simulink model "test_mdl_NI"  (R2018a)
settings: Solver=VariableStepAuto  StartTime=0.0  StopTime=10.0  RelTol=1e-3
(part 9 of 24)

== system test_mdl_NI/Subsystem/GWM/Body_Info_4_FD1_Ox242 ==
  in_port : Inport
  BattULo_I_Actl : Terminator
  BattULo_U_Actl : Terminator
  BrkTrnShifLck_B_Stat : Terminator
  DcacElPw_D_Rq : Terminator
  DriverCrankingReq : Terminator
  EngOff_T_Actl : Terminator
  FuelPumpPwr_D_Stat : Terminator
  PrkLckCtlAvail_T_Stat : Terminator
  PrkLckCtlMsgTxt_D_Rq : Terminator
  PrkLckCtlTow_B_Enbl : Terminator
  PrkLckCtlUnlck_D_Stat : Terminator
  PrkLckCtl_B_Enbl : Terminator
  PtLatchActv_B_RqBcm : Terminator
  ReFuelSwtchStat_D_Actl : Terminator
  bus_selector : BusSelector  OutputSignals=BattULo_I_Actl,BattULo_U_Actl,BrkTrnShifLck_B_Stat,DcacElPw_D_Rq,DriverCrankingReq,EngOff_T_Actl,FuelPumpPwr_D_Stat,PrkLckCtlAvail_T_Stat,PrkLckCtlMsgTxt_D_Rq,PrkLckCtlTow_B_Enbl,PrkLckCtlUnlck_D_Stat,PrkLckCtl_B_Enbl,PtLatchActv_B_RqBcm,ReFuelSwtchStat_D_Actl,immoSecureIdleMode
  immoSecureIdleMode : Terminator
  wires:
  in_port/1 -> bus_selector/1  "Body_Info_4_FD1_Ox242"
  bus_selector/1 -> BattULo_I_Actl/1  "<BattULo_I_Actl>"
  bus_selector/2 -> BattULo_U_Actl/1  "<BattULo_U_Actl>"
  bus_selector/3 -> BrkTrnShifLck_B_Stat/1  "<BrkTrnShifLck_B_Stat>"
  bus_selector/4 -> DcacElPw_D_Rq/1  "<DcacElPw_D_Rq>"
  bus_selector/5 -> DriverCrankingReq/1  "<DriverCrankingReq>"
  bus_selector/6 -> EngOff_T_Actl/1  "<EngOff_T_Actl>"
  bus_selector/7 -> FuelPumpPwr_D_Stat/1  "<FuelPumpPwr_D_Stat>"
  bus_selector/8 -> PrkLckCtlAvail_T_Stat/1  "<PrkLckCtlAvail_T_Stat>"
  bus_selector/9 -> PrkLckCtlMsgTxt_D_Rq/1  "<PrkLckCtlMsgTxt_D_Rq>"
  bus_selector/10 -> PrkLckCtlTow_B_Enbl/1  "<PrkLckCtlTow_B_Enbl>"
  bus_selector/11 -> PrkLckCtlUnlck_D_Stat/1  "<PrkLckCtlUnlck_D_Stat>"
  bus_selector/12 -> PrkLckCtl_B_Enbl/1  "<PrkLckCtl_B_Enbl>"
  bus_selector/13 -> PtLatchActv_B_RqBcm/1  "<PtLatchActv_B_RqBcm>"
  bus_selector/14 -> ReFuelSwtchStat_D_Actl/1  "<ReFuelSwtchStat_D_Actl>"
  bus_selector/15 -> immoSecureIdleMode/1  "<immoSecureIdleMode>"

== system test_mdl_NI/Subsystem/GWM/Body_Info_6_FD1_Ox38D ==
  in_port : Inport
  DrLatchMsgTxt_D_Rq : Terminator
  ElPwPoint_D_Rq : Terminator
  HeadLghtHiPrmsn_D_Stat : Terminator
  IgnPsswrdDsply_B_Rq : Terminator
  KeyAdmnTot_No_Cnt : Terminator
  KeyMykeyTot_No_Cnt : Terminator
  Keycode_Status : Terminator
  PEBackupSlot_Stats : Terminator
  PoliceIdlMde_D_Stat : Terminator
  PrmtrAlrmEvnt_D_Stat : Terminator
  PrsnlDevcChrgEnbl_B_Rq : Terminator
  SecurityMsgTxt_D_Rq : Terminator
  SteWhlLckMsgTxt_D_Rq : Terminator
  TracKeyMde_D_Stat : Terminator
  bus_selector : BusSelector  OutputSignals=DrLatchMsgTxt_D_Rq,ElPwPoint_D_Rq,HeadLghtHiPrmsn_D_Stat,IgnPsswrdDsply_B_Rq,KeyAdmnTot_No_Cnt,KeyMykeyTot_No_Cnt,Keycode_Status,PEBackupSlot_Stats,PoliceIdlMde_D_Stat,PrmtrAlrmEvnt_D_Stat,PrsnlDevcChrgEnbl_B_Rq,SecurityMsgTxt_D_Rq,SteWhlLckMsgTxt_D_Rq,TracKeyMde_D_Stat,immoMsgTxt_D_Rq
  immoMsgTxt_D_Rq : Terminator
  wires:
  in_port/1 -> bus_selector/1  "Body_Info_6_FD1_Ox38D"
  bus_selector/1 -> DrLatchMsgTxt_D_Rq/1  "<DrLatchMsgTxt_D_Rq>"
  bus_selector/2 -> ElPwPoint_D_Rq/1  "<ElPwPoint_D_Rq>"
  bus_selector/3 -> HeadLghtHiPrmsn_D_Stat/1  "<HeadLghtHiPrmsn_D_Stat>"
  bus_selector/4 -> IgnPsswrdDsply_B_Rq/1  "<IgnPsswrdDsply_B_Rq>"
  bus_selector/5 -> KeyAdmnTot_No_Cnt/1  "<KeyAdmnTot_No_Cnt>"
  bus_selector/6 -> KeyMykeyTot_No_Cnt/1  "<KeyMykeyTot_No_Cnt>"
  bus_selector/7 -> Keycode_Status/1  "<Keycode_Status>"
  bus_selector/8 -> PEBackupSlot_Stats/1  "<PEBackupSlot_Stats>"
  bus_selector/9 -> PoliceIdlMde_D_Stat/1  "<PoliceIdlMde_D_Stat>"
  bus_selector/10 -> PrmtrAlrmEvnt_D_Stat/1  "<PrmtrAlrmEvnt_D_Stat>"
  bus_selector/11 -> PrsnlDevcChrgEnbl_B_Rq/1  "<PrsnlDevcChrgEnbl_B_Rq>"
  bus_selector/12 -> SecurityMsgTxt_D_Rq/1  "<SecurityMsgTxt_D_Rq>"
  bus_selector/13 -> SteWhlLckMsgTxt_D_Rq/1  "<SteWhlLckMsgTxt_D_Rq>"
  bus_selector/14 -> TracKeyMde_D_Stat/1  "<TracKeyMde_D_Stat>"
  bus_selector/15 -> immoMsgTxt_D_Rq/1  "<immoMsgTxt_D_Rq>"

== system test_mdl_NI/Subsystem/GWM/Body_Info_8_FD1_Ox3B9 ==
  in_port : Inport
  BattRgenLoChrg_D_Rq : Terminator
  BattRgenLoDChrg_D_Rq : Terminator
  ChrgCordLck_B_Stat : Terminator
  ChrgCordResp1_No_Actl : Terminator
  ChrgCordResp2_No_Actl : Terminator
  WakeAlarm0_D_Stat : Terminator
  WakeAlarm1_D_Stat : Terminator
  WakeAlarm2_D_Stat : Terminator
  WakeAlarm3_D_Stat : Terminator
  bus_selector : BusSelector  OutputSignals=BattRgenLoChrg_D_Rq,BattRgenLoDChrg_D_Rq,ChrgCordLck_B_Stat,ChrgCordResp1_No_Actl,ChrgCordResp2_No_Actl,WakeAlarm0_D_Stat,WakeAlarm1_D_Stat,WakeAlarm2_D_Stat,WakeAlarm3_D_Stat
  wires:
  in_port/1 -> bus_selector/1  "Body_Info_8_FD1_Ox3B9"
  bus_selector/1 -> BattRgenLoChrg_D_Rq/1  "<BattRgenLoChrg_D_Rq>"
  bus_selector/2 -> BattRgenLoDChrg_D_Rq/1  "<BattRgenLoDChrg_D_Rq>"
  bus_selector/3 -> ChrgCordLck_B_Stat/1  "<ChrgCordLck_B_Stat>"
  bus_selector/4 -> ChrgCordResp1_No_Actl/1  "<ChrgCordResp1_No_Actl>"
  bus_selector/5 -> ChrgCordResp2_No_Actl/1  "<ChrgCordResp2_No_Actl>"
  bus_selector/6 -> WakeAlarm0_D_Stat/1  "<WakeAlarm0_D_Stat>"
  bus_selector/7 -> WakeAlarm1_D_Stat/1  "<WakeAlarm1_D_Stat>"
  bus_selector/8 -> WakeAlarm2_D_Stat/1  "<WakeAlarm2_D_Stat>"
  bus_selector/9 -> WakeAlarm3_D_Stat/1  "<WakeAlarm3_D_Stat>"

== system test_mdl_NI/Subsystem/GWM/Body_Info_9_FD1_Ox3A3 ==
  in_port : Inport
  AdvStrt_D_Stat : Terminator
  CrnkInhbt_B_Stat : Terminator
  CrnkInhbt_No_Cnt : Terminator
  CrnkInhbt_No_Cs : Terminator
  DrvInCtl_B_Stat : Terminator
  EngStrtActv_B_Stat : Terminator
  EngStrt_B_Rq : Terminator
  IgnPreOffActv_B_Stat : Terminator
  PtWakeReas_D_Stat : Terminator
  StrtrMtrCtlDStat_No_Cs : Terminator
  VehOnSrc_D_Stat : Terminator
  bus_selector : BusSelector  OutputSignals=AdvStrt_D_Stat,CrnkInhbt_B_Stat,CrnkInhbt_No_Cnt,CrnkInhbt_No_Cs,DrvInCtl_B_Stat,EngStrtActv_B_Stat,EngStrt_B_Rq,IgnPreOffActv_B_Stat,PtWakeReas_D_Stat,StrtrMtrCtlDStat_No_Cs,VehOnSrc_D_Stat
  wires:
  in_port/1 -> bus_selector/1  "Body_Info_9_FD1_Ox3A3"
  bus_selector/1 -> AdvStrt_D_Stat/1  "<AdvStrt_D_Stat>"
  bus_selector/2 -> CrnkInhbt_B_Stat/1  "<CrnkInhbt_B_Stat>"
  bus_selector/3 -> CrnkInhbt_No_Cnt/1  "<CrnkInhbt_No_Cnt>"
  bus_selector/4 -> CrnkInhbt_No_Cs/1  "<CrnkInhbt_No_Cs>"
  bus_selector/5 -> DrvInCtl_B_Stat/1  "<DrvInCtl_B_Stat>"
  bus_selector/6 -> EngStrtActv_B_Stat/1  "<EngStrtActv_B_Stat>"
  bus_selector/7 -> EngStrt_B_Rq/1  "<EngStrt_B_Rq>"
  bus_selector/8 -> IgnPreOffActv_B_Stat/1  "<IgnPreOffActv_B_Stat>"
  bus_selector/9 -> PtWakeReas_D_Stat/1  "<PtWakeReas_D_Stat>"
  bus_selector/10 -> StrtrMtrCtlDStat_No_Cs/1  "<StrtrMtrCtlDStat_No_Cs>"
  bus_selector/11 -> VehOnSrc_D_Stat/1  "<VehOnSrc_D_Stat>"

== system test_mdl_NI/Subsystem/GWM/Climate_Cntrl_Data_2_FD1_Ox35E ==
  in_port : Inport
  AutoStpHvacDelta_I_Est : Terminator
  CabnAmb_Te_Actl : Terminator
  ClimtThrmlLoad_No_Actl : Terminator
  HvacAir_Flw_Est : Terminator
  HvacBlwrFront_D_Stat : Terminator
  HvacRec_Pc_Est : Terminator
  HvacRemoteStrt_N_Rq : Terminator
  bus_selector : BusSelector  OutputSignals=AutoStpHvacDelta_I_Est,CabnAmb_Te_Actl,ClimtThrmlLoad_No_Actl,HvacAir_Flw_Est,HvacBlwrFront_D_Stat,HvacRec_Pc_Est,HvacRemoteStrt_N_Rq
  wires:
  in_port/1 -> bus_selector/1  "Climate_Cntrl_Data_2_FD1_Ox35E"
  bus_selector/1 -> AutoStpHvacDelta_I_Est/1  "<AutoStpHvacDelta_I_Est>"
  bus_selector/2 -> CabnAmb_Te_Actl/1  "<CabnAmb_Te_Actl>"
  bus_selector/3 -> ClimtThrmlLoad_No_Actl/1  "<ClimtThrmlLoad_No_Actl>"
  bus_selector/4 -> HvacAir_Flw_Est/1  "<HvacAir_Flw_Est>"
  bus_selector/5 -> HvacBlwrFront_D_Stat/1  "<HvacBlwrFront_D_Stat>"
  bus_selector/6 -> HvacRec_Pc_Est/1  "<HvacRec_Pc_Est>"
  bus_selector/7 -> HvacRemoteStrt_N_Rq/1  "<HvacRemoteStrt_N_Rq>"

== system test_mdl_NI/Subsystem/GWM/Climate_Control_Data_FD1_Ox41A ==
  in_port : Inport
  AutoHoldSwtch_D_Stat : Terminator
  LpdbDfrstRearOn_B_Rq : Terminator
  LpdbHeatWiprPrk_B_Rq : Terminator
  LpdbPtc1_B_Rq : Terminator
  LpdbPtc2_B_Rq : Terminator
  LpdbPtc3_B_Rq : Terminator
  MirrorHeatOn_B_Rq : Terminator
  Outside_Air_Temp_Stat : Terminator
  Remote_Start_QuietMode : Terminator
  SteWhlHeat_D_Rq : Terminator
  bus_selector : BusSelector  OutputSignals=AutoHoldSwtch_D_Stat,LpdbDfrstRearOn_B_Rq,LpdbHeatWiprPrk_B_Rq,LpdbPtc1_B_Rq,LpdbPtc2_B_Rq,LpdbPtc3_B_Rq,MirrorHeatOn_B_Rq,Outside_Air_Temp_Stat,Remote_Start_QuietMode,SteWhlHeat_D_Rq
  wires:
  in_port/1 -> bus_selector/1  "Climate_Control_Data_FD1_Ox41A"
  bus_selector/1 -> AutoHoldSwtch_D_Stat/1  "<AutoHoldSwtch_D_Stat>"
  bus_selector/2 -> LpdbDfrstRearOn_B_Rq/1  "<LpdbDfrstRearOn_B_Rq>"
  bus_selector/3 -> LpdbHeatWiprPrk_B_Rq/1  "<LpdbHeatWiprPrk_B_Rq>"
  bus_selector/4 -> LpdbPtc1_B_Rq/1  "<LpdbPtc1_B_Rq>"
  bus_selector/5 -> LpdbPtc2_B_Rq/1  "<LpdbPtc2_B_Rq>"
  bus_selector/6 -> LpdbPtc3_B_Rq/1  "<LpdbPtc3_B_Rq>"
  bus_selector/7 -> MirrorHeatOn_B_Rq/1  "<MirrorHeatOn_B_Rq>"
  bus_selector/8 -> Outside_Air_Temp_Stat/1  "<Outside_Air_Temp_Stat>"
  bus_selector/9 -> Remote_Start_QuietMode/1  "<Remote_Start_QuietMode>"
  bus_selector/10 -> SteWhlHeat_D_Rq/1  "<SteWhlHeat_D_Rq>"

== system test_mdl_NI/Subsystem/GWM/Cluster_HEV_Data8_FD1_Ox317 ==
  in_port : Inport
  ConsAvgTrip_Fe_Dsply : Terminator
  DrvEffLvl_No_Stat : Terminator
  EngAirFilt_B_RqReset : Terminator
  GpsElMdeSel_B_Rq : Terminator
  LongTermReset_B_Rq : Terminator
  bus_selector : BusSelector  OutputSignals=ConsAvgTrip_Fe_Dsply,DrvEffLvl_No_Stat,EngAirFilt_B_RqReset,GpsElMdeSel_B_Rq,LongTermReset_B_Rq
  wires:
  in_port/1 -> bus_selector/1  "Cluster_HEV_Data8_FD1_Ox317"
  bus_selector/1 -> ConsAvgTrip_Fe_Dsply/1  "<ConsAvgTrip_Fe_Dsply>"
  bus_selector/2 -> DrvEffLvl_No_Stat/1  "<DrvEffLvl_No_Stat>"
  bus_selector/3 -> EngAirFilt_B_RqReset/1  "<EngAirFilt_B_RqReset>"
  bus_selector/4 -> GpsElMdeSel_B_Rq/1  "<GpsElMdeSel_B_Rq>"
  bus_selector/5 -> LongTermReset_B_Rq/1  "<LongTermReset_B_Rq>"

== system test_mdl_NI/Subsystem/GWM/Cluster_Info1_FD1_Ox430 ==
  in_port : Inport
  AccDeny_B_RqIpc : Terminator
  AccEnbl_B_RqDrv : Terminator
  BulbChkActv_B_Stat : Terminator
  DrvSlipCtlMde_B_Rq2 : Terminator
  DrvSlipCtlMde_D_Rq : Terminator
  EngIdlShutDown_B_RqDrv : Terminator
  EngOilLife_B_RqReset : Terminator
  HaDsplyCpblty_B_Stat : Terminator
  HsaMde_D_Rq : Terminator
  KeyTypeChngMykey_D_Rq : Terminator
  LscmbbStat_B_Actl : Terminator
  ManRgen_D_Rq : Terminator
  MetricActv_B_Actl : Terminator
  NtrlTowMdeEnbl_B_RqDrv : Terminator
  OdometerMasterValue : Terminator
  ParkDetect_Stat : Terminator
  Power_Liftgate_Mode_Cmd : Terminator
  ReducedGuard_D_Rq : Terminator
  TRAILER_BRAKE_CONFIG : Terminator
  TRLR_SWAY_CONFIG_CMD : Terminator
  TrlrBrkMde_D_Rq : Terminator
  bus_selector : BusSelector  OutputSignals=AccDeny_B_RqIpc,AccEnbl_B_RqDrv,BulbChkActv_B_Stat,DrvSlipCtlMde_B_Rq2,DrvSlipCtlMde_D_Rq,EngIdlShutDown_B_RqDrv,EngOilLife_B_RqReset,HaDsplyCpblty_B_Stat,HsaMde_D_Rq,KeyTypeChngMykey_D_Rq,LscmbbStat_B_Actl,ManRgen_D_Rq,MetricActv_B_Actl,NtrlTowMdeEnbl_B_RqDrv,OdometerMasterValue,ParkDetect_Stat,Power_Liftgate_Mode_Cmd,ReducedGuard_D_Rq,TRAILER_BRAKE_CONFIG,TRLR_SWAY_CONFIG_CMD,TrlrBrkMde_D_Rq,ePRNDL_MODE
  ePRNDL_MODE : Terminator
  wires:
  in_port/1 -> bus_selector/1  "Cluster_Info1_FD1_Ox430"
  bus_selector/1 -> AccDeny_B_RqIpc/1  "<AccDeny_B_RqIpc>"
  bus_selector/2 -> AccEnbl_B_RqDrv/1  "<AccEnbl_B_RqDrv>"
  bus_selector/3 -> BulbChkActv_B_Stat/1  "<BulbChkActv_B_Stat>"
  bus_selector/4 -> DrvSlipCtlMde_B_Rq2/1  "<DrvSlipCtlMde_B_Rq2>"
  bus_selector/5 -> DrvSlipCtlMde_D_Rq/1  "<DrvSlipCtlMde_D_Rq>"
  bus_selector/6 -> EngIdlShutDown_B_RqDrv/1  "<EngIdlShutDown_B_RqDrv>"
  bus_selector/7 -> EngOilLife_B_RqReset/1  "<EngOilLife_B_RqReset>"
  bus_selector/8 -> HaDsplyCpblty_B_Stat/1  "<HaDsplyCpblty_B_Stat>"
  bus_selector/9 -> HsaMde_D_Rq/1  "<HsaMde_D_Rq>"
  bus_selector/10 -> KeyTypeChngMykey_D_Rq/1  "<KeyTypeChngMykey_D_Rq>"
  bus_selector/11 -> LscmbbStat_B_Actl/1  "<LscmbbStat_B_Actl>"
  bus_selector/12 -> ManRgen_D_Rq/1  "<ManRgen_D_Rq>"
  bus_selector/13 -> MetricActv_B_Actl/1  "<MetricActv_B_Actl>"
  bus_selector/14 -> NtrlTowMdeEnbl_B_RqDrv/1  "<NtrlTowMdeEnbl_B_RqDrv>"
  bus_selector/15 -> OdometerMasterValue/1  "<OdometerMasterValue>"
  bus_selector/16 -> ParkDetect_Stat/1  "<ParkDetect_Stat>"
  bus_selector/17 -> Power_Liftgate_Mode_Cmd/1  "<Power_Liftgate_Mode_Cmd>"
  bus_selector/18 -> ReducedGuard_D_Rq/1  "<ReducedGuard_D_Rq>"
  bus_selector/19 -> TRAILER_BRAKE_CONFIG/1  "<TRAILER_BRAKE_CONFIG>"
  bus_selector/20 -> TRLR_SWAY_CONFIG_CMD/1  "<TRLR_SWAY_CONFIG_CMD>"
  bus_selector/21 -> TrlrBrkMde_D_Rq/1  "<TrlrBrkMde_D_Rq>"
  bus_selector/22 -> ePRNDL_MODE/1  "<ePRNDL_MODE>"

== system test_mdl_NI/Subsystem/GWM/Cluster_Info_3_FD1_Ox434 ==
  in_port : Inport
  AutoRgen_D_Rq : Terminator
  DISPLAY_SPEED_OFFSET : Terminator
  DISPLAY_SPEED_SCALING : Terminator
  DrvSlipCtlMde_B_RqMyKey : Terminator
  FUEL_SENSOR_NUM : Terminator
  FuelLvlActvSide_No_Raw : Terminator
  FuelLvlPssvSide_No_Raw : Terminator
  FuelLvlWarn_D_Actl : Terminator
  FuelLvl_Pc_Dsply : Terminator
  FuelSecndActv_B_Actl : Terminator
  HILL_DESC_SW : Terminator
  OdoTripRx_B_Actl : Terminator
  Veh_V_CompLimMx : Terminator
  W2S_LAMP_OK : Terminator
  bus_selector : BusSelector  OutputSignals=AutoRgen_D_Rq,DISPLAY_SPEED_OFFSET,DISPLAY_SPEED_SCALING,DrvSlipCtlMde_B_RqMyKey,FUEL_SENSOR_NUM,FuelLvlActvSide_No_Raw,FuelLvlPssvSide_No_Raw,FuelLvlWarn_D_Actl,FuelLvl_Pc_Dsply,FuelSecndActv_B_Actl,HILL_DESC_SW,OdoTripRx_B_Actl,Veh_V_CompLimMx,W2S_LAMP_OK
  wires:
  in_port/1 -> bus_selector/1  "Cluster_Info_3_FD1_Ox434"
  bus_selector/1 -> AutoRgen_D_Rq/1  "<AutoRgen_D_Rq>"
  bus_selector/2 -> DISPLAY_SPEED_OFFSET/1  "<DISPLAY_SPEED_OFFSET>"
  bus_selector/3 -> DISPLAY_SPEED_SCALING/1  "<DISPLAY_SPEED_SCALING>"
  bus_selector/4 -> DrvSlipCtlMde_B_RqMyKey/1  "<DrvSlipCtlMde_B_RqMyKey>"
  bus_selector/5 -> FUEL_SENSOR_NUM/1  "<FUEL_SENSOR_NUM>"
  bus_selector/6 -> FuelLvlActvSide_No_Raw/1  "<FuelLvlActvSide_No_Raw>"
  bus_selector/7 -> FuelLvlPssvSide_No_Raw/1  "<FuelLvlPssvSide_No_Raw>"
  bus_selector/8 -> FuelLvlWarn_D_Actl/1  "<FuelLvlWarn_D_Actl>"
  bus_selector/9 -> FuelLvl_Pc_Dsply/1  "<FuelLvl_Pc_Dsply>"
  bus_selector/10 -> FuelSecndActv_B_Actl/1  "<FuelSecndActv_B_Actl>"
  bus_selector/11 -> HILL_DESC_SW/1  "<HILL_DESC_SW>"
  bus_selector/12 -> OdoTripRx_B_Actl/1  "<OdoTripRx_B_Actl>"
  bus_selector/13 -> Veh_V_CompLimMx/1  "<Veh_V_CompLimMx>"
  bus_selector/14 -> W2S_LAMP_OK/1  "<W2S_LAMP_OK>"

== system test_mdl_NI/Subsystem/GWM/Cluster_Lighting_Rq_FD1_Ox3C8 ==
  in_port : Inport
  IsaOffst_D_Rq : Terminator
  SlMde_D_Rq : Terminator
  bus_selector : BusSelector  OutputSignals=IsaOffst_D_Rq,SlMde_D_Rq
  wires:
  in_port/1 -> bus_selector/1  "Cluster_Lighting_Rq_FD1_Ox3C8"
  bus_selector/1 -> IsaOffst_D_Rq/1  "<IsaOffst_D_Rq>"
  bus_selector/2 -> SlMde_D_Rq/1  "<SlMde_D_Rq>"

== system test_mdl_NI/Subsystem/GWM/Compressor_Req_FD1_Ox326 ==
  in_port : Inport
  ClimtCool_D_Rq : Terminator
  ClimtHeat_D_Rq : Terminator
  ClimtPw_B_Rq : Terminator
  HvacAirCond_B_Rq : Terminator
  HvacEvap_Te_Actl : Terminator
  HvacEvap_Te_Offst : Terminator
  HvacEvap_Te_Rq : Terminator
  HvacHtrCore_Te_Rq : Terminator
  SnowPlowMde_B_Enbl : Terminator
  StopStrtDrvMde_B_RqBtn : Terminator
  bus_selector : BusSelector  OutputSignals=ClimtCool_D_Rq,ClimtHeat_D_Rq,ClimtPw_B_Rq,HvacAirCond_B_Rq,HvacEvap_Te_Actl,HvacEvap_Te_Offst,HvacEvap_Te_Rq,HvacHtrCore_Te_Rq,SnowPlowMde_B_Enbl,StopStrtDrvMde_B_RqBtn
  wires:
  in_port/1 -> bus_selector/1  "Compressor_Req_FD1_Ox326"
  bus_selector/1 -> ClimtCool_D_Rq/1  "<ClimtCool_D_Rq>"
  bus_selector/2 -> ClimtHeat_D_Rq/1  "<ClimtHeat_D_Rq>"
  bus_selector/3 -> ClimtPw_B_Rq/1  "<ClimtPw_B_Rq>"
  bus_selector/4 -> HvacAirCond_B_Rq/1  "<HvacAirCond_B_Rq>"
  bus_selector/5 -> HvacEvap_Te_Actl/1  "<HvacEvap_Te_Actl>"
  bus_selector/6 -> HvacEvap_Te_Offst/1  "<HvacEvap_Te_Offst>"
  bus_selector/7 -> HvacEvap_Te_Rq/1  "<HvacEvap_Te_Rq>"
  bus_selector/8 -> HvacHtrCore_Te_Rq/1  "<HvacHtrCore_Te_Rq>"
  bus_selector/9 -> SnowPlowMde_B_Enbl/1  "<SnowPlowMde_B_Enbl>"
  bus_selector/10 -> StopStrtDrvMde_B_RqBtn/1  "<StopStrtDrvMde_B_RqBtn>"

== system test_mdl_NI/Subsystem/GWM/CruiseCtrl_Strg_Data_FD1_Ox8B ==
  in_port : Inport
  AccButtnGapDecPress2 : Terminator
  AccButtnGapIncPress2 : Terminator
  AccButtnGpTogglePress2 : Terminator
  ActvFrontSteLck_D_Stat : Terminator
  ActvFrontSteMsgTxt_D_Rq : Terminator
  AfsPw_B_Rq : Terminator
  AslButtnOnOffCnclPres2 : Terminator
  AslButtnOnOffPress2 : Terminator
  CcAslButtnCnclPress2 : Terminator
  CcAslButtnCnclResPres2 : Terminator
  CcAslButtnDeny_B_Actl2 : Terminator
  CcAslButtnIndxDecPres2 : Terminator
  CcAslButtnIndxIncPres2 : Terminator
  CcAslButtnOffCnclPres2 : Terminator
  CcAslButtnOnOffCncl2 : Terminator
  CcAslButtnOnPress2 : Terminator
  CcAslButtnResDecPress2 : Terminator
  CcAslButtnResIncPress2 : Terminator
  CcAslButtnSetDecPress2 : Terminator
  CcAslButtnSetIncPress2 : Terminator
  CcAslButtnSetPress2 : Terminator
  CcAsllButtnResPress2 : Terminator
  CcButtnOffPress2 : Terminator
  CcButtnOnOffCnclPress2 : Terminator
  CcButtnOnOffPress2 : Terminator
  CcButtnOnPress2 : Terminator
  SelDrvMdeAdptSte_D_Stat : Terminator
  TjaButtnOnOffPress2 : Terminator
  bus_selector : BusSelector  OutputSignals=AccButtnGapDecPress2,AccButtnGapIncPress2,AccButtnGpTogglePress2,ActvFrontSteLck_D_Stat,ActvFrontSteMsgTxt_D_Rq,AfsPw_B_Rq,AslButtnOnOffCnclPres2,AslButtnOnOffPress2,CcAslButtnCnclPress2,CcAslButtnCnclResPres2,CcAslButtnDeny_B_Actl2,CcAslButtnIndxDecPres2,CcAslButtnIndxIncPres2,CcAslButtnOffCnclPres2,CcAslButtnOnOffCncl2,CcAslButtnOnPress2,CcAslButtnResDecPress2,CcAslButtnResIncPress2,CcAslButtnSetDecPress2,CcAslButtnSetIncPress2,CcAslButtnSetPress2,CcAsllButtnResPress2,CcButtnOffPress2,CcButtnOnOffCnclPress2,CcButtnOnOffPress2,CcButtnOnPress2,SelDrvMdeAdptSte_D_Stat,TjaButtnOnOffPress2
  wires:
  in_port/1 -> bus_selector/1  "CruiseCtrl_Strg_Data_FD1_Ox8B"
  bus_selector/1 -> AccButtnGapDecPress2/1  "<AccButtnGapDecPress2>"
  bus_selector/2 -> AccButtnGapIncPress2/1  "<AccButtnGapIncPress2>"
  bus_selector/3 -> AccButtnGpTogglePress2/1  "<AccButtnGpTogglePress2>"
  bus_selector/4 -> ActvFrontSteLck_D_Stat/1  "<ActvFrontSteLck_D_Stat>"
  bus_selector/5 -> ActvFrontSteMsgTxt_D_Rq/1  "<ActvFrontSteMsgTxt_D_Rq>"
  bus_selector/6 -> AfsPw_B_Rq/1  "<AfsPw_B_Rq>"
  bus_selector/7 -> AslButtnOnOffCnclPres2/1  "<AslButtnOnOffCnclPres2>"
  bus_selector/8 -> AslButtnOnOffPress2/1  "<AslButtnOnOffPress2>"
  bus_selector/9 -> CcAslButtnCnclPress2/1  "<CcAslButtnCnclPress2>"
  bus_selector/10 -> CcAslButtnCnclResPres2/1  "<CcAslButtnCnclResPres2>"
  bus_selector/11 -> CcAslButtnDeny_B_Actl2/1  "<CcAslButtnDeny_B_Actl2>"
  bus_selector/12 -> CcAslButtnIndxDecPres2/1  "<CcAslButtnIndxDecPres2>"
  bus_selector/13 -> CcAslButtnIndxIncPres2/1  "<CcAslButtnIndxIncPres2>"
  bus_selector/14 -> CcAslButtnOffCnclPres2/1  "<CcAslButtnOffCnclPres2>"
  bus_selector/15 -> CcAslButtnOnOffCncl2/1  "<CcAslButtnOnOffCncl2>"
  bus_selector/16 -> CcAslButtnOnPress2/1  "<CcAslButtnOnPress2>"
  bus_selector/17 -> CcAslButtnResDecPress2/1  "<CcAslButtnResDecPress2>"
  bus_selector/18 -> CcAslButtnResIncPress2/1  "<CcAslButtnResIncPress2>"
  bus_selector/19 -> CcAslButtnSetDecPress2/1  "<CcAslButtnSetDecPress2>"
  bus_selector/20 -> CcAslButtnSetIncPress2/1  "<CcAslButtnSetIncPress2>"
  bus_selector/21 -> CcAslButtnSetPress2/1  "<CcAslButtnSetPress2>"
  bus_selector/22 -> CcAsllButtnResPress2/1  "<CcAsllButtnResPress2>"
  bus_selector/23 -> CcButtnOffPress2/1  "<CcButtnOffPress2>"
  bus_selector/24 -> CcButtnOnOffCnclPress2/1  "<CcButtnOnOffCnclPress2>"
  bus_selector/25 -> CcButtnOnOffPress2/1  "<CcButtnOnOffPress2>"
  bus_selector/26 -> CcButtnOnPress2/1  "<CcButtnOnPress2>"
  bus_selector/27 -> SelDrvMdeAdptSte_D_Stat/1  "<SelDrvMdeAdptSte_D_Stat>"
  bus_selector/28 -> TjaButtnOnOffPress2/1  "<TjaButtnOnOffPress2>"

== system test_mdl_NI/Subsystem/GWM/DCACA_Data1_FD1_Ox39A ==
  in_port : Inport
  CoolFanDcac_D_Rq : Terminator
  DcacAcUDetct_B_Falt : Terminator
  DcacBp1BrkrOpn_B_Falt : Terminator
  DcacBp2BrkrOpn_B_Falt : Terminator
  DcacClntFlw_D_Rq : Terminator
  DcacErr_B_Stat : Terminator
  DcacGfci_B_Falt : Terminator
  DcacIpRcBrkrOpn_B_Falt : Terminator
  DcacOverTe_B_Falt : Terminator
  DcacOvrld_B_Falt : Terminator
  DcacPlugPrsnt_B_Stat : Terminator
  DcacRdy_D2_Stat : Terminator
  DcacRdy_D_Stat : Terminator
  bus_selector : BusSelector  OutputSignals=CoolFanDcac_D_Rq,DcacAcUDetct_B_Falt,DcacBp1BrkrOpn_B_Falt,DcacBp2BrkrOpn_B_Falt,DcacClntFlw_D_Rq,DcacErr_B_Stat,DcacGfci_B_Falt,DcacIpRcBrkrOpn_B_Falt,DcacOverTe_B_Falt,DcacOvrld_B_Falt,DcacPlugPrsnt_B_Stat,DcacRdy_D2_Stat,DcacRdy_D_Stat
  wires:
  in_port/1 -> bus_selector/1  "DCACA_Data1_FD1_Ox39A"
  bus_selector/1 -> CoolFanDcac_D_Rq/1  "<CoolFanDcac_D_Rq>"
  bus_selector/2 -> DcacAcUDetct_B_Falt/1  "<DcacAcUDetct_B_Falt>"
  bus_selector/3 -> DcacBp1BrkrOpn_B_Falt/1  "<DcacBp1BrkrOpn_B_Falt>"
  bus_selector/4 -> DcacBp2BrkrOpn_B_Falt/1  "<DcacBp2BrkrOpn_B_Falt>"
  bus_selector/5 -> DcacClntFlw_D_Rq/1  "<DcacClntFlw_D_Rq>"
  bus_selector/6 -> DcacErr_B_Stat/1  "<DcacErr_B_Stat>"
  bus_selector/7 -> DcacGfci_B_Falt/1  "<DcacGfci_B_Falt>"
  bus_selector/8 -> DcacIpRcBrkrOpn_B_Falt/1  "<DcacIpRcBrkrOpn_B_Falt>"
  bus_selector/9 -> DcacOverTe_B_Falt/1  "<DcacOverTe_B_Falt>"
  bus_selector/10 -> DcacOvrld_B_Falt/1  "<DcacOvrld_B_Falt>"
  bus_selector/11 -> DcacPlugPrsnt_B_Stat/1  "<DcacPlugPrsnt_B_Stat>"
  bus_selector/12 -> DcacRdy_D2_Stat/1  "<DcacRdy_D2_Stat>"
  bus_selector/13 -> DcacRdy_D_Stat/1  "<DcacRdy_D_Stat>"

== system test_mdl_NI/Subsystem/GWM/DCACA_Data2_FD1_Ox39B ==
  in_port : Inport
  DcacIn_I_Actl : Terminator
  DcacIn_U2_Actl : Terminator
  DcacIn_U_Actl : Terminator
  Dcac_Te_Actl : Terminator
  bus_selector : BusSelector  OutputSignals=DcacIn_I_Actl,DcacIn_U2_Actl,DcacIn_U_Actl,Dcac_Te_Actl
  wires:
  in_port/1 -> bus_selector/1  "DCACA_Data2_FD1_Ox39B"
  bus_selector/1 -> DcacIn_I_Actl/1  "<DcacIn_I_Actl>"
  bus_selector/2 -> DcacIn_U2_Actl/1  "<DcacIn_U2_Actl>"
  bus_selector/3 -> DcacIn_U_Actl/1  "<DcacIn_U_Actl>"
  bus_selector/4 -> Dcac_Te_Actl/1  "<Dcac_Te_Actl>"

== system test_mdl_NI/Subsystem/GWM/DCACA_Data3_FD1_Ox39C ==
  in_port : Inport
  DcacIn_Pw_Mx : Terminator
  DcacOut1_Pw_Actl : Terminator
  DcacOut2_Pw_Actl : Terminator
  DcacOut_Pw_Mx : Terminator
  bus_selector : BusSelector  OutputSignals=DcacIn_Pw_Mx,DcacOut1_Pw_Actl,DcacOut2_Pw_Actl,DcacOut_Pw_Mx
  wires:
  in_port/1 -> bus_selector/1  "DCACA_Data3_FD1_Ox39C"
  bus_selector/1 -> DcacIn_Pw_Mx/1  "<DcacIn_Pw_Mx>"
  bus_selector/2 -> DcacOut1_Pw_Actl/1  "<DcacOut1_Pw_Actl>"
  bus_selector/3 -> DcacOut2_Pw_Actl/1  "<DcacOut2_Pw_Actl>"
  bus_selector/4 -> DcacOut_Pw_Mx/1  "<DcacOut_Pw_Mx>"

== system test_mdl_NI/Subsystem/GWM/DTE_ECGtoHPCM_Ox338 ==
  in_port : Inport
  DteCldBattULo_Eff_Actl : Terminator
  DteCldClimt_Eff_Actl : Terminator
  DteCldDcac_B_Stat : Terminator
  DteCldDrv_Eff_Actl : Terminator
  DteCldExtTe_B_Stat : Terminator
  DteCldExt_Eff_Actl : Terminator
  DteCldId_No_Actl : Terminator
  DteCldPayload_B_Stat : Terminator
  DteCldRoute_B_Stat : Terminator
  DteCldTerrain_B_Stat : Terminator
  DteCldTraffic_B_Stat : Terminator
  DteCldTrip_L_Actl : Terminator
  DteCldTrlrOff_B_Stat : Terminator
  DteCldTrlrOn_B_Stat : Terminator
  bus_selector : BusSelector  OutputSignals=DteCldBattULo_Eff_Actl,DteCldClimt_Eff_Actl,DteCldDcac_B_Stat,DteCldDrv_Eff_Actl,DteCldExtTe_B_Stat,DteCldExt_Eff_Actl,DteCldId_No_Actl,DteCldPayload_B_Stat,DteCldRoute_B_Stat,DteCldTerrain_B_Stat,DteCldTraffic_B_Stat,DteCldTrip_L_Actl,DteCldTrlrOff_B_Stat,DteCldTrlrOn_B_Stat
  wires:
  in_port/1 -> bus_selector/1  "DTE_ECGtoHPCM_Ox338"
  bus_selector/1 -> DteCldBattULo_Eff_Actl/1  "<DteCldBattULo_Eff_Actl>"
  bus_selector/2 -> DteCldClimt_Eff_Actl/1  "<DteCldClimt_Eff_Actl>"
  bus_selector/3 -> DteCldDcac_B_Stat/1  "<DteCldDcac_B_Stat>"
  bus_selector/4 -> DteCldDrv_Eff_Actl/1  "<DteCldDrv_Eff_Actl>"
  bus_selector/5 -> DteCldExtTe_B_Stat/1  "<DteCldExtTe_B_Stat>"
  bus_selector/6 -> DteCldExt_Eff_Actl/1  "<DteCldExt_Eff_Actl>"
  bus_selector/7 -> DteCldId_No_Actl/1  "<DteCldId_No_Actl>"
  bus_selector/8 -> DteCldPayload_B_Stat/1  "<DteCldPayload_B_Stat>"
  bus_selector/9 -> DteCldRoute_B_Stat/1  "<DteCldRoute_B_Stat>"
  bus_selector/10 -> DteCldTerrain_B_Stat/1  "<DteCldTerrain_B_Stat>"
  bus_selector/11 -> DteCldTraffic_B_Stat/1  "<DteCldTraffic_B_Stat>"
  bus_selector/12 -> DteCldTrip_L_Actl/1  "<DteCldTrip_L_Actl>"
  bus_selector/13 -> DteCldTrlrOff_B_Stat/1  "<DteCldTrlrOff_B_Stat>"
  bus_selector/14 -> DteCldTrlrOn_B_Stat/1  "<DteCldTrlrOn_B_Stat>"

== system test_mdl_NI/Subsystem/GWM/Driver_Dr_Stat_FD1_Ox332 ==
  in_port : Inport
  BLISLEDStatDriverSide : Terminator
  ChildLckFdbckRd_B_Stat : Terminator
  ChildLckPw_D_Rq : Terminator
  ChildLckPw_N_Cnt : Terminator
  Driver_Lock_Sw_Cnt : Terminator
  Driver_Lock_Sw_Stat : Terminator
  KeyCylSwDrvDr_D_Stat : Terminator
  RollCodeDrvDrKeyCyl : Terminator
  RvrseMirrorChime_B_Rq : Terminator
  WndwDrvSide_D_Stat : Terminator
  bus_selector : BusSelector  OutputSignals=BLISLEDStatDriverSide,ChildLckFdbckRd_B_Stat,ChildLckPw_D_Rq,ChildLckPw_N_Cnt,Driver_Lock_Sw_Cnt,Driver_Lock_Sw_Stat,KeyCylSwDrvDr_D_Stat,RollCodeDrvDrKeyCyl,RvrseMirrorChime_B_Rq,WndwDrvSide_D_Stat
  wires:
  in_port/1 -> bus_selector/1  "Driver_Dr_Stat_FD1_Ox332"
  bus_selector/1 -> BLISLEDStatDriverSide/1  "<BLISLEDStatDriverSide>"
  bus_selector/2 -> ChildLckFdbckRd_B_Stat/1  "<ChildLckFdbckRd_B_Stat>"
  bus_selector/3 -> ChildLckPw_D_Rq/1  "<ChildLckPw_D_Rq>"
  bus_selector/4 -> ChildLckPw_N_Cnt/1  "<ChildLckPw_N_Cnt>"
  bus_selector/5 -> Driver_Lock_Sw_Cnt/1  "<Driver_Lock_Sw_Cnt>"
  bus_selector/6 -> Driver_Lock_Sw_Stat/1  "<Driver_Lock_Sw_Stat>"
  bus_selector/7 -> KeyCylSwDrvDr_D_Stat/1  "<KeyCylSwDrvDr_D_Stat>"
  bus_selector/8 -> RollCodeDrvDrKeyCyl/1  "<RollCodeDrvDrKeyCyl>"
  bus_selector/9 -> RvrseMirrorChime_B_Rq/1  "<RvrseMirrorChime_B_Rq>"
  bus_selector/10 -> WndwDrvSide_D_Stat/1  "<WndwDrvSide_D_Stat>"

== system test_mdl_NI/Subsystem/GWM/Dsp_Request_Signals11_FD1_Ox192 ==
  in_port : Inport
  ApaMdeStat_D_RqDrv : Terminator
  ApaSwtch_D_RqMnu : Terminator
  CamAutoTowbarZoom : Terminator
  CamraOvrlDyn_D_Rq : Terminator
  CamraOvrlStat_D_Rq : Terminator
  CamraViewSplit_B_Rq : Terminator
  CamraZoomMan_D_Rq : Terminator
  DistanceBarSetting : Terminator
  PrkAidSwtch_D_RqMnu : Terminator
  bus_selector : BusSelector  OutputSignals=ApaMdeStat_D_RqDrv,ApaSwtch_D_RqMnu,CamAutoTowbarZoom,CamraOvrlDyn_D_Rq,CamraOvrlStat_D_Rq,CamraViewSplit_B_Rq,CamraZoomMan_D_Rq,DistanceBarSetting,PrkAidSwtch_D_RqMnu
  wires:
  in_port/1 -> bus_selector/1  "Dsp_Request_Signals11_FD1_Ox192"
  bus_selector/1 -> ApaMdeStat_D_RqDrv/1  "<ApaMdeStat_D_RqDrv>"
  bus_selector/2 -> ApaSwtch_D_RqMnu/1  "<ApaSwtch_D_RqMnu>"
  bus_selector/3 -> CamAutoTowbarZoom/1  "<CamAutoTowbarZoom>"
  bus_selector/4 -> CamraOvrlDyn_D_Rq/1  "<CamraOvrlDyn_D_Rq>"
  bus_selector/5 -> CamraOvrlStat_D_Rq/1  "<CamraOvrlStat_D_Rq>"
  bus_selector/6 -> CamraViewSplit_B_Rq/1  "<CamraViewSplit_B_Rq>"
  bus_selector/7 -> CamraZoomMan_D_Rq/1  "<CamraZoomMan_D_Rq>"
  bus_selector/8 -> DistanceBarSetting/1  "<DistanceBarSetting>"
  bus_selector/9 -> PrkAidSwtch_D_RqMnu/1  "<PrkAidSwtch_D_RqMnu>"

== system test_mdl_NI/Subsystem/GWM/ECG_Data2_FD1_Ox488 ==
  in_port : Inport
  DataMntrSustn_B_Rq : Terminator
  DgtlCommPncReset_B_Req : Terminator
  PwSustnRdata_B_RqTelem : Terminator
  bus_selector : BusSelector  OutputSignals=DataMntrSustn_B_Rq,DgtlCommPncReset_B_Req,PwSustnRdata_B_RqTelem
  wires:
  in_port/1 -> bus_selector/1  "ECG_Data2_FD1_Ox488"
  bus_selector/1 -> DataMntrSustn_B_Rq/1  "<DataMntrSustn_B_Rq>"
  bus_selector/2 -> DgtlCommPncReset_B_Req/1  "<DgtlCommPncReset_B_Req>"
  bus_selector/3 -> PwSustnRdata_B_RqTelem/1  "<PwSustnRdata_B_RqTelem>"

== system test_mdl_NI/Subsystem/GWM/ECG_Data3_FD1_Ox375 ==
  in_port : Inport
  BattULoChrg_D_RqOta : Terminator
  CanMsg375_No_Cnt : Terminator
  CanMsg375_No_Crc : Terminator
  OtaActv_D_Stat : Terminator
  VehOnRqstr_D_Stat : Terminator
  VehOn_D_RqCld : Terminator
  VehStrtInhbt_D_Dsply : Terminator
  VehStrtInhbt_D_RqCld : Terminator
  VehStrtInhbt_T_Dsply : Terminator
  bus_selector : BusSelector  OutputSignals=BattULoChrg_D_RqOta,CanMsg375_No_Cnt,CanMsg375_No_Crc,OtaActv_D_Stat,VehOnRqstr_D_Stat,VehOn_D_RqCld,VehStrtInhbt_D_Dsply,VehStrtInhbt_D_RqCld,VehStrtInhbt_T_Dsply
  wires:
  in_port/1 -> bus_selector/1  "ECG_Data3_FD1_Ox375"
  bus_selector/1 -> BattULoChrg_D_RqOta/1  "<BattULoChrg_D_RqOta>"
  bus_selector/2 -> CanMsg375_No_Cnt/1  "<CanMsg375_No_Cnt>"
  bus_selector/3 -> CanMsg375_No_Crc/1  "<CanMsg375_No_Crc>"
  bus_selector/4 -> OtaActv_D_Stat/1  "<OtaActv_D_Stat>"
  bus_selector/5 -> VehOnRqstr_D_Stat/1  "<VehOnRqstr_D_Stat>"
  bus_selector/6 -> VehOn_D_RqCld/1  "<VehOn_D_RqCld>"
  bus_selector/7 -> VehStrtInhbt_D_Dsply/1  "<VehStrtInhbt_D_Dsply>"
  bus_selector/8 -> VehStrtInhbt_D_RqCld/1  "<VehStrtInhbt_D_RqCld>"
  bus_selector/9 -> VehStrtInhbt_T_Dsply/1  "<VehStrtInhbt_T_Dsply>"

== system test_mdl_NI/Subsystem/GWM/ECG_Data4_FD1_Ox226 ==
  in_port : Inport
  PtWakeupActv1_B_Rq : Terminator
  bus_selector : BusSelector  OutputSignals=PtWakeupActv1_B_Rq
  wires:
  in_port/1 -> bus_selector/1  "ECG_Data4_FD1_Ox226"
  bus_selector/1 -> PtWakeupActv1_B_Rq/1  "<PtWakeupActv1_B_Rq>"

== system test_mdl_NI/Subsystem/GWM/ECG_Data_FD1_Ox32A ==
  in_port : Inport
  ChrgrPncEnbl_D_Rq : Terminator
  ChrgrPncSustn_B_Rq : Terminator
  ExtLghtDsply_B_StatArb : Terminator
  ExtLghtFront_D_RqOta : Terminator
  ExtLghtLeft_D_RqOta : Terminator
  ExtLghtRear_D_RqOta : Terminator
  ExtLghtRight_D_RqOta : Terminator
  NtfyDrvSocLvl1_Pc_Rq : Terminator
  NtfyDrvTrgtDist_L_Rq : Terminator
  OBCCSerial_D_Rq : Terminator
  PtRmtRprt_D_Stat : Terminator
  TlghtTest_D_RqArb : Terminator
  bus_selector : BusSelector  OutputSignals=ChrgrPncEnbl_D_Rq,ChrgrPncSustn_B_Rq,ExtLghtDsply_B_StatArb,ExtLghtFront_D_RqOta,ExtLghtLeft_D_RqOta,ExtLghtRear_D_RqOta,ExtLghtRight_D_RqOta,NtfyDrvSocLvl1_Pc_Rq,NtfyDrvTrgtDist_L_Rq,OBCCSerial_D_Rq,PtRmtRprt_D_Stat,TlghtTest_D_RqArb
  wires:
  in_port/1 -> bus_selector/1  "ECG_Data_FD1_Ox32A"
  bus_selector/1 -> ChrgrPncEnbl_D_Rq/1  "<ChrgrPncEnbl_D_Rq>"
  bus_selector/2 -> ChrgrPncSustn_B_Rq/1  "<ChrgrPncSustn_B_Rq>"
  bus_selector/3 -> ExtLghtDsply_B_StatArb/1  "<ExtLghtDsply_B_StatArb>"
  bus_selector/4 -> ExtLghtFront_D_RqOta/1  "<ExtLghtFront_D_RqOta>"
  bus_selector/5 -> ExtLghtLeft_D_RqOta/1  "<ExtLghtLeft_D_RqOta>"
  bus_selector/6 -> ExtLghtRear_D_RqOta/1  "<ExtLghtRear_D_RqOta>"
  bus_selector/7 -> ExtLghtRight_D_RqOta/1  "<ExtLghtRight_D_RqOta>"
  bus_selector/8 -> NtfyDrvSocLvl1_Pc_Rq/1  "<NtfyDrvSocLvl1_Pc_Rq>"
  bus_selector/9 -> NtfyDrvTrgtDist_L_Rq/1  "<NtfyDrvTrgtDist_L_Rq>"
  bus_selector/10 -> OBCCSerial_D_Rq/1  "<OBCCSerial_D_Rq>"
  bus_selector/11 -> PtRmtRprt_D_Stat/1  "<PtRmtRprt_D_Stat>"
  bus_selector/12 -> TlghtTest_D_RqArb/1  "<TlghtTest_D_RqArb>"

== system test_mdl_NI/Subsystem/GWM/ElecHorizon_Data1_FD1_Ox22E ==
  in_port : Inport
  EhData1_No_Actl : Terminator
  bus_selector : BusSelector  OutputSignals=EhData1_No_Actl
  wires:
  in_port/1 -> bus_selector/1  "ElecHorizon_Data1_FD1_Ox22E"
  bus_selector/1 -> EhData1_No_Actl/1  "<EhData1_No_Actl>"

== system test_mdl_NI/Subsystem/GWM/ElecHorizon_Data2_FD1_Ox22F ==
  in_port : Inport
  EhData2_No_Actl : Terminator
  bus_selector : BusSelector  OutputSignals=EhData2_No_Actl
  wires:
  in_port/1 -> bus_selector/1  "ElecHorizon_Data2_FD1_Ox22F"
  bus_selector/1 -> EhData2_No_Actl/1  "<EhData2_No_Actl>"

== system test_mdl_NI/Subsystem/GWM/FourByFourSwitchData_FD1_Ox460 ==
  in_port : Inport
  AwdMde_D_RqDrv : Terminator
  DrvSlipCtlMde_B_Rq3 : Terminator
  HdcSwtchPos_B_Actl : Terminator
  HybMdeSwtch_B_Rq : Terminator
  RearDiffLck_D_RqDrv : Terminator
  TrailCtlSwtch_B_Stat3 : Terminator
  bus_selector : BusSelector  OutputSignals=AwdMde_D_RqDrv,DrvSlipCtlMde_B_Rq3,HdcSwtchPos_B_Actl,HybMdeSwtch_B_Rq,RearDiffLck_D_RqDrv,TrailCtlSwtch_B_Stat3
  wires:
  in_port/1 -> bus_selector/1  "FourByFourSwitchData_FD1_Ox460"
  bus_selector/1 -> AwdMde_D_RqDrv/1  "<AwdMde_D_RqDrv>"
  bus_selector/2 -> DrvSlipCtlMde_B_Rq3/1  "<DrvSlipCtlMde_B_Rq3>"
  bus_selector/3 -> HdcSwtchPos_B_Actl/1  "<HdcSwtchPos_B_Actl>"
  bus_selector/4 -> HybMdeSwtch_B_Rq/1  "<HybMdeSwtch_B_Rq>"
  bus_selector/5 -> RearDiffLck_D_RqDrv/1  "<RearDiffLck_D_RqDrv>"
  bus_selector/6 -> TrailCtlSwtch_B_Stat3/1  "<TrailCtlSwtch_B_Stat3>"

== system test_mdl_NI/Subsystem/GWM/GGCC_Config_Mgmt_ID_1_FD1_Ox40A ==
  in_port : Inport
  VehicleGGCCData : Terminator
  bus_selector : BusSelector  OutputSignals=VehicleGGCCData
  wires:
  in_port/1 -> bus_selector/1  "GGCC_Config_Mgmt_ID_1_FD1_Ox40A"
  bus_selector/1 -> VehicleGGCCData/1  "<VehicleGGCCData>"

== system test_mdl_NI/Subsystem/GWM/GWM_AutoSar_NetMgmt_FD1_Ox59E ==
  in_port : Inport
  GWM_AutoSarNMControl : Terminator
  GWM_AutoSarNMNodeId : Terminator
  GWM_AutoSarNMReserved{1..4} (4 alike) : Terminator
  GWM_GWNMProxy : Terminator
  GWM_GWOnBoardTester : Terminator
  bus_selector : BusSelector  OutputSignals=GWM_AutoSarNMControl,GWM_AutoSarNMNodeId,GWM_AutoSarNMReserved1,GWM_AutoSarNMReserved2,GWM_AutoSarNMReserved3,GWM_AutoSarNMReserved4,GWM_GWNMProxy,GWM_GWOnBoardTester
  wires:
  in_port/1 -> bus_selector/1  "GWM_AutoSar_NetMgmt_FD1_Ox59E"
  bus_selector/1 -> GWM_AutoSarNMControl/1  "<GWM_AutoSarNMControl>"
  bus_selector/2 -> GWM_AutoSarNMNodeId/1  "<GWM_AutoSarNMNodeId>"
  bus_selector/3 -> GWM_AutoSarNMReserved1/1  "<GWM_AutoSarNMReserved1>"
  bus_selector/4 -> GWM_AutoSarNMReserved2/1  "<GWM_AutoSarNMReserved2>"
  bus_selector/5 -> GWM_AutoSarNMReserved3/1  "<GWM_AutoSarNMReserved3>"
  bus_selector/6 -> GWM_AutoSarNMReserved4/1  "<GWM_AutoSarNMReserved4>"
  bus_selector/7 -> GWM_GWNMProxy/1  "<GWM_GWNMProxy>"
  bus_selector/8 -> GWM_GWOnBoardTester/1  "<GWM_GWOnBoardTester>"

== system test_mdl_NI/Subsystem/GWM/Gear_Shift_by_Wire_2_FD1_Ox168 ==
  in_port : Inport
  GearButtnStuck_B_Actl : Terminator
  GsmSrvcRqd_B_Rq : Terminator
  TrnGearPwmFalt_B_Actl : Terminator
  bus_selector : BusSelector  OutputSignals=GearButtnStuck_B_Actl,GsmSrvcRqd_B_Rq,TrnGearPwmFalt_B_Actl
  wires:
  in_port/1 -> bus_selector/1  "Gear_Shift_by_Wire_2_FD1_Ox168"
  bus_selector/1 -> GearButtnStuck_B_Actl/1  "<GearButtnStuck_B_Actl>"
  bus_selector/2 -> GsmSrvcRqd_B_Rq/1  "<GsmSrvcRqd_B_Rq>"
  bus_selector/3 -> TrnGearPwmFalt_B_Actl/1  "<TrnGearPwmFalt_B_Actl>"

== system test_mdl_NI/Subsystem/GWM/Gear_Shift_by_Wire_FD1_Ox5A ==
  in_port : Inport
  BrkSwtchPos_B_ActlGsm : Terminator
  DrQltyDrv_D_StatGsm : Terminator
  GsmGearMsgTxt_D_Rq : Terminator
  PrkBrkActv_D_RqGsmGear : Terminator
  TrnBtsiOvrrd_B_Stat : Terminator
  TrnGearButtn_B_ActlD0 : Terminator
  TrnGearButtn_B_ActlD1 : Terminator
  TrnGearButtn_B_ActlD2 : Terminator
  TrnGearButtn_B_ActlM0 : Terminator
  TrnGearButtn_B_ActlM1 : Terminator
  TrnGearButtn_B_ActlM2 : Terminator
  TrnGearButtn_B_ActlN0 : Terminator
  TrnGearButtn_B_ActlN1 : Terminator
  TrnGearButtn_B_ActlN2 : Terminator
  TrnGearButtn_B_ActlP0 : Terminator
  TrnGearButtn_B_ActlP1 : Terminator
  TrnGearButtn_B_ActlP2 : Terminator
  TrnGearButtn_B_ActlR0 : Terminator
  TrnGearButtn_B_ActlR1 : Terminator
  TrnGearButtn_B_ActlR2 : Terminator
  TrnGearButtn_U_Actl : Terminator
  TrnGearRqCnt_B_Actl : Terminator
  TrnGear_D_RqDrv : Terminator
  TrnGear_No_Cnt : Terminator
  TrnGear_No_Cs : Terminator
  TrnGsmNtmState_D_Actl : Terminator
  TrnRng_D_RqGsm : Terminator
  TrnValidGearRq_D_Stat : Terminator
  bus_selector : BusSelector  OutputSignals=BrkSwtchPos_B_ActlGsm,DrQltyDrv_D_StatGsm,GsmGearMsgTxt_D_Rq,PrkBrkActv_D_RqGsmGear,TrnBtsiOvrrd_B_Stat,TrnGearButtn_B_ActlD0,TrnGearButtn_B_ActlD1,TrnGearButtn_B_ActlD2,TrnGearButtn_B_ActlM0,TrnGearButtn_B_ActlM1,TrnGearButtn_B_ActlM2,TrnGearButtn_B_ActlN0,TrnGearButtn_B_ActlN1,TrnGearButtn_B_ActlN2,TrnGearButtn_B_ActlP0,TrnGearButtn_B_ActlP1,TrnGearButtn_B_ActlP2,TrnGearButtn_B_ActlR0,TrnGearButtn_B_ActlR1,TrnGearButtn_B_ActlR2,TrnGearButtn_U_Actl,TrnGearRqCnt_B_Actl,TrnGear_D_RqDrv,TrnGear_No_Cnt,TrnGear_No_Cs,TrnGsmNtmState_D_Actl,TrnRng_D_RqGsm,TrnValidGearRq_D_Stat
  wires:
  in_port/1 -> bus_selector/1  "Gear_Shift_by_Wire_FD1_Ox5A"
  bus_selector/1 -> BrkSwtchPos_B_ActlGsm/1  "<BrkSwtchPos_B_ActlGsm>"
  bus_selector/2 -> DrQltyDrv_D_StatGsm/1  "<DrQltyDrv_D_StatGsm>"
  bus_selector/3 -> GsmGearMsgTxt_D_Rq/1  "<GsmGearMsgTxt_D_Rq>"
  bus_selector/4 -> PrkBrkActv_D_RqGsmGear/1  "<PrkBrkActv_D_RqGsmGear>"
  bus_selector/5 -> TrnBtsiOvrrd_B_Stat/1  "<TrnBtsiOvrrd_B_Stat>"
  bus_selector/6 -> TrnGearButtn_B_ActlD0/1  "<TrnGearButtn_B_ActlD0>"
  bus_selector/7 -> TrnGearButtn_B_ActlD1/1  "<TrnGearButtn_B_ActlD1>"
  bus_selector/8 -> TrnGearButtn_B_ActlD2/1  "<TrnGearButtn_B_ActlD2>"
  bus_selector/9 -> TrnGearButtn_B_ActlM0/1  "<TrnGearButtn_B_ActlM0>"
  bus_selector/10 -> TrnGearButtn_B_ActlM1/1  "<TrnGearButtn_B_ActlM1>"
  bus_selector/11 -> TrnGearButtn_B_ActlM2/1  "<TrnGearButtn_B_ActlM2>"
  bus_selector/12 -> TrnGearButtn_B_ActlN0/1  "<TrnGearButtn_B_ActlN0>"
  bus_selector/13 -> TrnGearButtn_B_ActlN1/1  "<TrnGearButtn_B_ActlN1>"
  bus_selector/14 -> TrnGearButtn_B_ActlN2/1  "<TrnGearButtn_B_ActlN2>"
  bus_selector/15 -> TrnGearButtn_B_ActlP0/1  "<TrnGearButtn_B_ActlP0>"
  bus_selector/16 -> TrnGearButtn_B_ActlP1/1  "<TrnGearButtn_B_ActlP1>"
  bus_selector/17 -> TrnGearButtn_B_ActlP2/1  "<TrnGearButtn_B_ActlP2>"
  bus_selector/18 -> TrnGearButtn_B_ActlR0/1  "<TrnGearButtn_B_ActlR0>"
  bus_selector/19 -> TrnGearButtn_B_ActlR1/1  "<TrnGearButtn_B_ActlR1>"
  bus_selector/20 -> TrnGearButtn_B_ActlR2/1  "<TrnGearButtn_B_ActlR2>"
  bus_selector/21 -> TrnGearButtn_U_Actl/1  "<TrnGearButtn_U_Actl>"
  bus_selector/22 -> TrnGearRqCnt_B_Actl/1  "<TrnGearRqCnt_B_Actl>"
  bus_selector/23 -> TrnGear_D_RqDrv/1  "<TrnGear_D_RqDrv>"
  bus_selector/24 -> TrnGear_No_Cnt/1  "<TrnGear_No_Cnt>"
  bus_selector/25 -> TrnGear_No_Cs/1  "<TrnGear_No_Cs>"
  bus_selector/26 -> TrnGsmNtmState_D_Actl/1  "<TrnGsmNtmState_D_Actl>"
  bus_selector/27 -> TrnRng_D_RqGsm/1  "<TrnRng_D_RqGsm>"
  bus_selector/28 -> TrnValidGearRq_D_Stat/1  "<TrnValidGearRq_D_Stat>"

== system test_mdl_NI/Subsystem/GWM/GlobalClock_Data_FD1_Ox84 ==
  in_port : Inport
  GlblClkDay_No_Actl : Terminator
  GlblClkHr_No_Actl : Terminator
  GlblClkMnte_No_Actl : Terminator
  GlblClkScnd_No_Actl : Terminator
  GlblClkYr_No_Actl : Terminator
  bus_selector : BusSelector  OutputSignals=GlblClkDay_No_Actl,GlblClkHr_No_Actl,GlblClkMnte_No_Actl,GlblClkScnd_No_Actl,GlblClkYr_No_Actl
  wires:
  in_port/1 -> bus_selector/1  "GlobalClock_Data_FD1_Ox84"
  bus_selector/1 -> GlblClkDay_No_Actl/1  "<GlblClkDay_No_Actl>"
  bus_selector/2 -> GlblClkHr_No_Actl/1  "<GlblClkHr_No_Actl>"
  bus_selector/3 -> GlblClkMnte_No_Actl/1  "<GlblClkMnte_No_Actl>"
  bus_selector/4 -> GlblClkScnd_No_Actl/1  "<GlblClkScnd_No_Actl>"
  bus_selector/5 -> GlblClkYr_No_Actl/1  "<GlblClkYr_No_Actl>"

== system test_mdl_NI/Subsystem/GWM/Global_PATS_Cntrl_Info_FD1_Ox41 ==
  in_port : Inport
  bus_selector : BusSelector  OutputSignals=immoControlCmd_T1,immoControlData_T1
  immoControlCmd_T1 : Terminator
  immoControlData_T1 : Terminator
  wires:
  in_port/1 -> bus_selector/1  "Global_PATS_Cntrl_Info_FD1_Ox41"
  bus_selector/1 -> immoControlCmd_T1/1  "<immoControlCmd_T1>"
  bus_selector/2 -> immoControlData_T1/1  "<immoControlData_T1>"

== system test_mdl_NI/Subsystem/GWM/Global_PATS_Ctrl_Info2_FD1_Ox42 ==
  in_port : Inport
  bus_selector : BusSelector  OutputSignals=immoControlCmd_T2,immoControlData_T2
  immoControlCmd_T2 : Terminator
  immoControlData_T2 : Terminator
  wires:
  in_port/1 -> bus_selector/1  "Global_PATS_Ctrl_Info2_FD1_Ox42"
  bus_selector/1 -> immoControlCmd_T2/1  "<immoControlCmd_T2>"
  bus_selector/2 -> immoControlData_T2/1  "<immoControlData_T2>"

== system test_mdl_NI/Subsystem/GWM/HeadUpDisplayReq_FD1_Ox18B ==
  in_port : Inport
  SelDrvMdeCnfm_D_Stat : Terminator
  bus_selector : BusSelector  OutputSignals=SelDrvMdeCnfm_D_Stat
  wires:
  in_port/1 -> bus_selector/1  "HeadUpDisplayReq_FD1_Ox18B"
  bus_selector/1 -> SelDrvMdeCnfm_D_Stat/1  "<SelDrvMdeCnfm_D_Stat>"

== system test_mdl_NI/Subsystem/GWM/IPC_Infotainment_FD1_Ox225 ==
  in_port : Inport
  BeltminderAudioMute : Terminator
  Chime_Source : Terminator
  HdcOn_B_Rq : Terminator
  IPC_Attn_Info_Audio : Terminator
  IPC_MyKeyVolLimit_St : Terminator
  IPC_New_Attn_Event : Terminator
  Power_Up_Chime_Modules : Terminator
  Veh_V2_Dsply : Terminator
  bus_selector : BusSelector  OutputSignals=BeltminderAudioMute,Chime_Source,HdcOn_B_Rq,IPC_Attn_Info_Audio,IPC_MyKeyVolLimit_St,IPC_New_Attn_Event,Power_Up_Chime_Modules,Veh_V2_Dsply
  wires:
  in_port/1 -> bus_selector/1  "IPC_Infotainment_FD1_Ox225"
  bus_selector/1 -> BeltminderAudioMute/1  "<BeltminderAudioMute>"
  bus_selector/2 -> Chime_Source/1  "<Chime_Source>"
  bus_selector/3 -> HdcOn_B_Rq/1  "<HdcOn_B_Rq>"
  bus_selector/4 -> IPC_Attn_Info_Audio/1  "<IPC_Attn_Info_Audio>"
  bus_selector/5 -> IPC_MyKeyVolLimit_St/1  "<IPC_MyKeyVolLimit_St>"
  bus_selector/6 -> IPC_New_Attn_Event/1  "<IPC_New_Attn_Event>"
  bus_selector/7 -> Power_Up_Chime_Modules/1  "<Power_Up_Chime_Modules>"
  bus_selector/8 -> Veh_V2_Dsply/1  "<Veh_V2_Dsply>"

== system test_mdl_NI/Subsystem/GWM/IPC_Send_Signals_2_FD1_Ox318 ==
  in_port : Inport
  ElLongTerm_L_Dsply : Terminator
  ElTrip_L_Dsply : Terminator
  FuelRange_L_Dsply : Terminator
  bus_selector : BusSelector  OutputSignals=ElLongTerm_L_Dsply,ElTrip_L_Dsply,FuelRange_L_Dsply
  wires:
  in_port/1 -> bus_selector/1  "IPC_Send_Signals_2_FD1_Ox318"
  bus_selector/1 -> ElLongTerm_L_Dsply/1  "<ElLongTerm_L_Dsply>"
  bus_selector/2 -> ElTrip_L_Dsply/1  "<ElTrip_L_Dsply>"
  bus_selector/3 -> FuelRange_L_Dsply/1  "<FuelRange_L_Dsply>"

== system test_mdl_NI/Subsystem/GWM/LocationServices_3_FD1_Ox21E ==
  in_port : Inport
  LocationServices_3 : Terminator
  bus_selector : BusSelector  OutputSignals=LocationServices_3
  wires:
  in_port/1 -> bus_selector/1  "LocationServices_3_FD1_Ox21E"
  bus_selector/1 -> LocationServices_3/1  "<LocationServices_3>"

== system test_mdl_NI/Subsystem/GWM/LocationServices_Data1_FD1_Ox47E ==
  in_port : Inport
  LocationServices_1 : Terminator
  bus_selector : BusSelector  OutputSignals=LocationServices_1
  wires:
  in_port/1 -> bus_selector/1  "LocationServices_Data1_FD1_Ox47E"
  bus_selector/1 -> LocationServices_1/1  "<LocationServices_1>"

== system test_mdl_NI/Subsystem/GWM/Locking_Systems_2_FD1_Ox331 ==
  in_port : Inport
  ChildLckMde_B_Stat : Terminator
  ChildLck_D_Dsply : Terminator
  DrTgateExtSwMde_B_Stat : Terminator
  DrTgateOpen_B_Rq : Terminator
  FobComm_D_Stat : Terminator
  Keyfob_Pad_Msg_Count : Terminator
  L_Pwr_Sliding_Dr_Rqst : Terminator
  LockInhibit : Terminator
  Lockmsgtxt_D_Rq : Terminator
  Power_Decklid_Rqst : Terminator
  Power_Liftgate_Rqst : Terminator
  R_Pwr_Sliding_Dr_Rqst : Terminator
  Remote_Device_Feedback : Terminator
  RollCodeUnlock : Terminator
  VehLckInd_D_Rq : Terminator
  Veh_Lock_EvNum : Terminator
  Veh_Lock_Requestor : Terminator
  Veh_Lock_Status : Terminator
  Veh_Lock_Sub_Id : Terminator
  WindowLockout_B_Stat : Terminator
  bus_selector : BusSelector  OutputSignals=ChildLckMde_B_Stat,ChildLck_D_Dsply,DrTgateExtSwMde_B_Stat,DrTgateOpen_B_Rq,FobComm_D_Stat,Keyfob_Pad_Msg_Count,L_Pwr_Sliding_Dr_Rqst,LockInhibit,Lockmsgtxt_D_Rq,Power_Decklid_Rqst,Power_Liftgate_Rqst,R_Pwr_Sliding_Dr_Rqst,Remote_Device_Feedback,RollCodeUnlock,VehLckInd_D_Rq,Veh_Lock_EvNum,Veh_Lock_Requestor,Veh_Lock_Status,Veh_Lock_Sub_Id,WindowLockout_B_Stat
  wires:
  in_port/1 -> bus_selector/1  "Locking_Systems_2_FD1_Ox331"
  bus_selector/1 -> ChildLckMde_B_Stat/1  "<ChildLckMde_B_Stat>"
  bus_selector/2 -> ChildLck_D_Dsply/1  "<ChildLck_D_Dsply>"
  bus_selector/3 -> DrTgateExtSwMde_B_Stat/1  "<DrTgateExtSwMde_B_Stat>"
  bus_selector/4 -> DrTgateOpen_B_Rq/1  "<DrTgateOpen_B_Rq>"
  bus_selector/5 -> FobComm_D_Stat/1  "<FobComm_D_Stat>"
  bus_selector/6 -> Keyfob_Pad_Msg_Count/1  "<Keyfob_Pad_Msg_Count>"
  bus_selector/7 -> L_Pwr_Sliding_Dr_Rqst/1  "<L_Pwr_Sliding_Dr_Rqst>"
  bus_selector/8 -> LockInhibit/1  "<LockInhibit>"
  bus_selector/9 -> Lockmsgtxt_D_Rq/1  "<Lockmsgtxt_D_Rq>"
  bus_selector/10 -> Power_Decklid_Rqst/1  "<Power_Decklid_Rqst>"
  bus_selector/11 -> Power_Liftgate_Rqst/1  "<Power_Liftgate_Rqst>"
  bus_selector/12 -> R_Pwr_Sliding_Dr_Rqst/1  "<R_Pwr_Sliding_Dr_Rqst>"
  bus_selector/13 -> Remote_Device_Feedback/1  "<Remote_Device_Feedback>"
  bus_selector/14 -> RollCodeUnlock/1  "<RollCodeUnlock>"
  bus_selector/15 -> VehLckInd_D_Rq/1  "<VehLckInd_D_Rq>"
  bus_selector/16 -> Veh_Lock_EvNum/1  "<Veh_Lock_EvNum>"
  bus_selector/17 -> Veh_Lock_Requestor/1  "<Veh_Lock_Requestor>"
  bus_selector/18 -> Veh_Lock_Status/1  "<Veh_Lock_Status>"
  bus_selector/19 -> Veh_Lock_Sub_Id/1  "<Veh_Lock_Sub_Id>"
  bus_selector/20 -> WindowLockout_B_Stat/1  "<WindowLockout_B_Stat>"

== system test_mdl_NI/Subsystem/GWM/MasterReset_HS3_ECGDat_FD1_Ox233 ==
  in_port : Inport
  DrvBhavWarn_B_Rq : Terminator
  FactoryReset_St : Terminator
  KeyOffPwMde_D_Stat : Terminator
  ModemReset_D_Stat : Terminator
  OfbChrgSetSync_D_Rq : Terminator
  bus_selector : BusSelector  OutputSignals=DrvBhavWarn_B_Rq,FactoryReset_St,KeyOffPwMde_D_Stat,ModemReset_D_Stat,OfbChrgSetSync_D_Rq
  wires:
  in_port/1 -> bus_selector/1  "MasterReset_HS3_ECGDat_FD1_Ox233"
  bus_selector/1 -> DrvBhavWarn_B_Rq/1  "<DrvBhavWarn_B_Rq>"
  bus_selector/2 -> FactoryReset_St/1  "<FactoryReset_St>"
  bus_selector/3 -> KeyOffPwMde_D_Stat/1  "<KeyOffPwMde_D_Stat>"
  bus_selector/4 -> ModemReset_D_Stat/1  "<ModemReset_D_Stat>"
  bus_selector/5 -> OfbChrgSetSync_D_Rq/1  "<OfbChrgSetSync_D_Rq>"

== system test_mdl_NI/Subsystem/GWM/Mc_Send_Signals_2_FD1_Ox2FD ==
  in_port : Inport
  AwdRnge_D_ActlIpc : Terminator
  BalrMde_D_Rq : Terminator
  BalrSwtch_D_Stat : Terminator
  BttOn_B_Rq : Terminator
  Btt_L_Actl : Terminator
  DrvInputRequired_B_Rq : Terminator
  EdmSailMde_B_RqDrv : Terminator
  EngExhMdeQuiet_D2_Rq : Terminator
  EsaOn_B_Rq : Terminator
  Mc_VehLangUsrSel_St : Terminator
  Mc_VehTimeFrmtUsrSel_St : Terminator
  Mc_VehUnitTempUsrSel_St : Terminator
  Mc_VehUntTrpCoUsrSel_St : Terminator
  Running_Board_Cmd : Terminator
  SelDrvMdeDsply_B_Avail : Terminator
  SelDrvMdeTxtReset_B_Rq : Terminator
  WaitToStartLamp_D_Falt : Terminator
  bus_selector : BusSelector  OutputSignals=AwdRnge_D_ActlIpc,BalrMde_D_Rq,BalrSwtch_D_Stat,BttOn_B_Rq,Btt_L_Actl,DrvInputRequired_B_Rq,EdmSailMde_B_RqDrv,EngExhMdeQuiet_D2_Rq,EsaOn_B_Rq,Mc_VehLangUsrSel_St,Mc_VehTimeFrmtUsrSel_St,Mc_VehUnitTempUsrSel_St,Mc_VehUntTrpCoUsrSel_St,Running_Board_Cmd,SelDrvMdeDsply_B_Avail,SelDrvMdeTxtReset_B_Rq,WaitToStartLamp_D_Falt
  wires:
  in_port/1 -> bus_selector/1  "Mc_Send_Signals_2_FD1_Ox2FD"
  bus_selector/1 -> AwdRnge_D_ActlIpc/1  "<AwdRnge_D_ActlIpc>"
  bus_selector/2 -> BalrMde_D_Rq/1  "<BalrMde_D_Rq>"
  bus_selector/3 -> BalrSwtch_D_Stat/1  "<BalrSwtch_D_Stat>"
  bus_selector/4 -> BttOn_B_Rq/1  "<BttOn_B_Rq>"
  bus_selector/5 -> Btt_L_Actl/1  "<Btt_L_Actl>"
  bus_selector/6 -> DrvInputRequired_B_Rq/1  "<DrvInputRequired_B_Rq>"
  bus_selector/7 -> EdmSailMde_B_RqDrv/1  "<EdmSailMde_B_RqDrv>"
  bus_selector/8 -> EngExhMdeQuiet_D2_Rq/1  "<EngExhMdeQuiet_D2_Rq>"
  bus_selector/9 -> EsaOn_B_Rq/1  "<EsaOn_B_Rq>"
  bus_selector/10 -> Mc_VehLangUsrSel_St/1  "<Mc_VehLangUsrSel_St>"
  bus_selector/11 -> Mc_VehTimeFrmtUsrSel_St/1  "<Mc_VehTimeFrmtUsrSel_St>"
  bus_selector/12 -> Mc_VehUnitTempUsrSel_St/1  "<Mc_VehUnitTempUsrSel_St>"
  bus_selector/13 -> Mc_VehUntTrpCoUsrSel_St/1  "<Mc_VehUntTrpCoUsrSel_St>"
  bus_selector/14 -> Running_Board_Cmd/1  "<Running_Board_Cmd>"
  bus_selector/15 -> SelDrvMdeDsply_B_Avail/1  "<SelDrvMdeDsply_B_Avail>"
  bus_selector/16 -> SelDrvMdeTxtReset_B_Rq/1  "<SelDrvMdeTxtReset_B_Rq>"
  bus_selector/17 -> WaitToStartLamp_D_Falt/1  "<WaitToStartLamp_D_Falt>"

== system test_mdl_NI/Subsystem/GWM/OTAFuncGWM_ECG_FD1_Ox1B9FFCD8 ==
  in_port : Inport
  OTAFuncGWM_ECG : Terminator
  bus_selector : BusSelector  OutputSignals=OTAFuncGWM_ECG
  wires:
  in_port/1 -> bus_selector/1  "OTAFuncGWM_ECG_FD1_Ox1B9FFCD8"
  bus_selector/1 -> OTAFuncGWM_ECG/1  "<OTAFuncGWM_ECG>"

== system test_mdl_NI/Subsystem/GWM/OTAPhysGWM_ECGtoABS_Ox1B90A0D8 ==
  in_port : Inport
  OTAPhysGWM_ECGtoABS : Terminator
  bus_selector : BusSelector  OutputSignals=OTAPhysGWM_ECGtoABS
  wires:
  in_port/1 -> bus_selector/1  "OTAPhysGWM_ECGtoABS_Ox1B90A0D8"
  bus_selector/1 -> OTAPhysGWM_ECGtoABS/1  "<OTAPhysGWM_ECGtoABS>"

== system test_mdl_NI/Subsystem/GWM/OTAPhysGWM_ECGtoCCM_Ox1B9054D8 ==
  in_port : Inport
  OTAPhysGWM_ECGtoCCM : Terminator
  bus_selector : BusSelector  OutputSignals=OTAPhysGWM_ECGtoCCM
  wires:
  in_port/1 -> bus_selector/1  "OTAPhysGWM_ECGtoCCM_Ox1B9054D8"
  bus_selector/1 -> OTAPhysGWM_ECGtoCCM/1  "<OTAPhysGWM_ECGtoCCM>"

== system test_mdl_NI/Subsystem/GWM/OTAPhysGWM_ECGtoIPMA_Ox1B9084D8 ==
  in_port : Inport
  OTAPhysGWM_ECGtoIPMA : Terminator
  bus_selector : BusSelector  OutputSignals=OTAPhysGWM_ECGtoIPMA
  wires:
  in_port/1 -> bus_selector/1  "OTAPhysGWM_ECGtoIPMA_Ox1B9084D8"
  bus_selector/1 -> OTAPhysGWM_ECGtoIPMA/1  "<OTAPhysGWM_ECGtoIPMA>"

== system test_mdl_NI/Subsystem/GWM/OTAPhysGWM_ECGtoPCM_Ox1B9040D8 ==
  in_port : Inport
  OTAPhysGWM_ECGtoPCM : Terminator
  bus_selector : BusSelector  OutputSignals=OTAPhysGWM_ECGtoPCM
  wires:
  in_port/1 -> bus_selector/1  "OTAPhysGWM_ECGtoPCM_Ox1B9040D8"
  bus_selector/1 -> OTAPhysGWM_ECGtoPCM/1  "<OTAPhysGWM_ECGtoPCM>"

== system test_mdl_NI/Subsystem/GWM/OTAPhysGWM_ECGtoSOBDMC_FD1_Ox1B9044D8 ==
  in_port : Inport
  OTAPhysGWM_ECGtoHPCM : Terminator
  bus_selector : BusSelector  OutputSignals=OTAPhysGWM_ECGtoHPCM
  wires:
  in_port/1 -> bus_selector/1  "OTAPhysGWM_ECGtoSOBDMC_FD1_Ox1B9044D8"
  bus_selector/1 -> OTAPhysGWM_ECGtoHPCM/1  "<OTAPhysGWM_ECGtoHPCM>"
